simulink model "pendulo"  (R2013a)
settings: Solver=ode5  StartTime=0.0  StopTime=100  FixedStep=.001  RelTol=1e-3
settings Model: Creator=Daniel  LastModifiedBy=Daniel

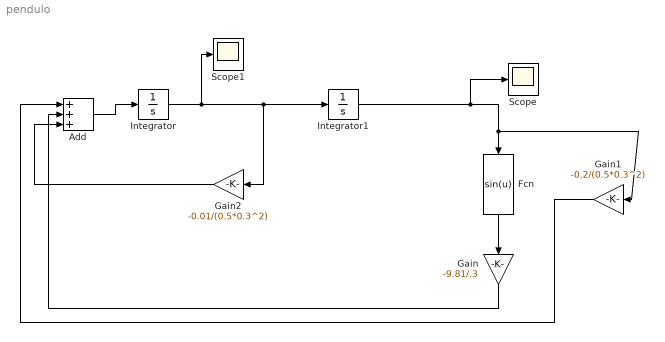
== system pendulo ==
  Add : Sum  Inputs=+++
  Fcn : Fcn  Expr=sin(u)
  Gain : Gain  Gain=-9.81/.3
  Gain1 : Gain  Gain=-0.2/(0.5*0.3^2)
  Gain2 : Gain  Gain=-0.01/(0.5*0.3^2)
  Integrator : Integrator
  Integrator1 : Integrator  InitialCondition=pi
  Scope : Scope
      settings: YMin=3.05  YMax=3.0825
  Scope1 : Scope
      settings: YMin=-1.75  YMax=1.75
  wires:
  Integrator/1 -> Scope1/1, Gain2/1, Integrator1/1
  Add/1 -> Integrator/1
  Fcn/1 -> Gain/1
  Gain/1 -> Add/2
  Integrator1/1 -> Scope/1, Gain1/1, Fcn/1
  Gain2/1 -> Add/3
  Gain1/1 -> Add/1
